simulink model "PID"  (R2021a)
settings: Solver=VariableStepAuto  StartTime=0.0  StopTime=20  RelTol=1e-3
settings Model: Creator=santiago  LastModifiedBy=santiago

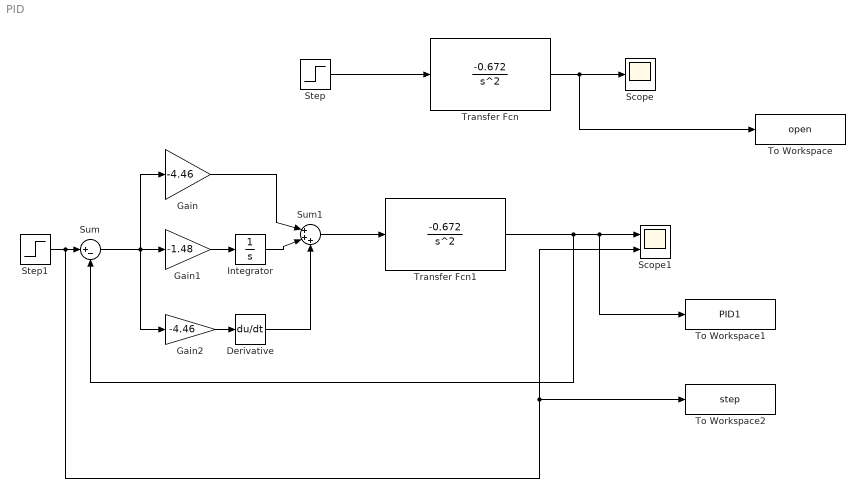
== system PID ==
  Derivative : Derivative
  Gain : Gain  Gain=-4.46
  Gain1 : Gain  Gain=-1.48
  Gain2 : Gain  Gain=-4.46
  Integrator : Integrator
  Scope : Scope
  Scope1 : Scope  NumInputPorts=2
  Step : Step  SampleTime=0
  Step1 : Step  SampleTime=0
  Sum : Sum  Inputs=|+-
  Sum1 : Sum  Inputs=|+++
  To Workspace : ToWorkspace  VariableName=open  SaveFormat=Timeseries  SampleTime=-1
  To Workspace1 : ToWorkspace  VariableName=PID1  SaveFormat=Timeseries  SampleTime=-1
  To Workspace2 : ToWorkspace  VariableName=step  SaveFormat=Timeseries  SampleTime=-1
  Transfer Fcn : TransferFcn  Numerator=[-0.672]  Denominator=[1 0 0]  ParameterTunability=Unconstrained
  Transfer Fcn1 : TransferFcn  Numerator=[-0.672]  Denominator=[1 0 0]  ParameterTunability=Unconstrained
  wires:
  Step/1 -> Transfer Fcn/1
  Transfer Fcn/1 -> To Workspace/1, Scope/1
  Gain/1 -> Sum1/1
  Sum/1 -> Gain2/1, Gain/1, Gain1/1
  Gain1/1 -> Integrator/1
  Integrator/1 -> Sum1/2
  Gain2/1 -> Derivative/1
  Derivative/1 -> Sum1/3
  Sum1/1 -> Transfer Fcn1/1
  Transfer Fcn1/1 -> Sum/2, To Workspace1/1, Scope1/1
  Step1/1 -> Sum/1, To Workspace2/1, Scope1/2
